simulink model "FUZZY_deg_neurospora_model_leloup"  (R2015a)
settings: Solver=ode4  StartTime=0.0  StopTime=72  FixedStep=0.01  RelTol=1e-3
values from neighbouring files (symbols this model uses):
  daynight_on = 0    [ALL_neurospora_init.m]    (also in ALL_neurospora_sim_run.m; FUZZY_deg_neurospora_init.m; FUZZY_deg_neurospora_sim_run.m; FUZZY_tsc_neurospora_init.m)
  k_1 = 0.5    [ALL_neurospora_init.m]    (also in FUZZY_deg_neurospora_init.m; FUZZY_tsc_neurospora_init.m; FUZZY_tsc_tsl_neurospora_init.m; FUZZY_tsl_neurospora_init.m)
  k_2 = 0.6    [ALL_neurospora_init.m]    (also in FUZZY_deg_neurospora_init.m; FUZZY_tsc_neurospora_init.m; FUZZY_tsc_tsl_neurospora_init.m; FUZZY_tsl_neurospora_init.m)
  K_I = 1    [ALL_neurospora_init.m]    (also in FUZZY_deg_neurospora_init.m; FUZZY_tsc_neurospora_init.m; FUZZY_tsc_tsl_neurospora_init.m; FUZZY_tsl_neurospora_init.m)
  k_s = 0.5    [ALL_neurospora_init.m]    (also in FUZZY_deg_neurospora_init.m; FUZZY_tsc_neurospora_init.m; FUZZY_tsc_tsl_neurospora_init.m; FUZZY_tsl_neurospora_init.m)
  n = 4    [ALL_neurospora_init.m]    (also in FUZZY_deg_neurospora_init.m; FUZZY_tsc_neurospora_init.m; FUZZY_tsc_tsl_neurospora_init.m; FUZZY_tsl_neurospora_init.m)
libraries: fuzblock x2
settings Model: Creator=jureb  LastModifiedBy=jureb

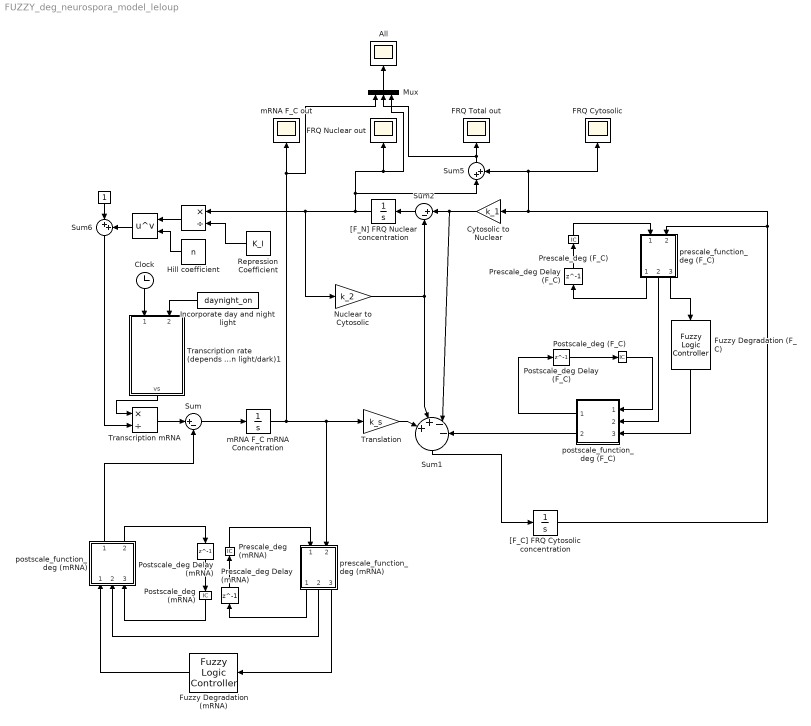
== system FUZZY_deg_neurospora_model_leloup ==
  " " : Math  Operator=pow  SaturateOnIntegerOverflow=on
  " " : Product  Inputs=*/
  "          " : Constant
  All : Scope
      settings: TimeRange=71.999776  YMin=0  YMax=9  SaveName=All
  Clock : Clock
  Cytosolic to Nuclear : Gain  Gain=k_1
  FRQ Cytosolic : Scope
      settings: TimeRange=71.999776  YMin=0.5  YMax=10  SaveName=F_C2
  FRQ Nuclear out : Scope
      settings: TimeRange=71.999776  YMin=0  YMax=4.5  SaveName=F_N
  FRQ Total out : Scope
      settings: TimeRange=71.999776  YMin=0.5  YMax=10  SaveName=F_FL_deg
  Fuzzy Degradation (F_C) : fuzblock/Fuzzy Logic  Controller  fis=deg
  Fuzzy Degradation (mRNA) : fuzblock/Fuzzy Logic  Controller  fis=deg
  Hill coefficient : Constant  Value=n
  Incorporate day and night light : Constant  Value=daynight_on
  Mux : Mux  Inputs=3
  Nuclear to Cytosolic : Gain  Gain=k_2
  Postscale_deg (F_C) : InitialCondition  Value=2
  Postscale_deg (mRNA) : InitialCondition  Value=0.5
  Postscale_deg Delay (F_C) : Delay  DelayLength=1  InitialCondition=1
  Postscale_deg Delay (mRNA) : Delay  DelayLength=1  InitialCondition=1
  Prescale_deg (F_C) : InitialCondition  Value=4
  Prescale_deg (mRNA) : InitialCondition  Value=4
  Prescale_deg Delay (F_C) : Delay  DelayLength=1  InitialCondition=1  UseCircularBuffer=on
  Prescale_deg Delay (mRNA) : Delay  DelayLength=1  InitialCondition=1  UseCircularBuffer=on
  Repression Coefficient : Constant  Value=K_I
  Sum : Sum  Inputs=|+-
  Sum1 : Sum  Inputs=|+|+|-|-
  Sum2 : Sum  Inputs=|+-
  Sum5 : Sum  Inputs=|++
  Sum6 : Sum  Inputs=|++
  Transcription mRNA : Product  Inputs=*/
  Transcription rate (depends on light/dark)1 : MATLAB Function  TreatAsAtomicUnit=on
  Translation : Gain  Gain=k_s
  "[F_C] FRQ Cytosolic concentration " : Integrator  InitialCondition=1
  "[F_N] FRQ Nuclear concentration" : Integrator  InitialCondition=1
  mRNA F_C mRNA Concentration : Integrator  InitialCondition=1  LowerSaturationLimit=0
  mRNA F_C out : Scope
      settings: TimeRange=71.999776  YMin=0  YMax=6  SaveName=mRNA
  postscale_function_deg (F_C) : MATLAB Function  TreatAsAtomicUnit=on
  postscale_function_deg (mRNA) : MATLAB Function  TreatAsAtomicUnit=on
  prescale_function_deg (F_C) : MATLAB Function  TreatAsAtomicUnit=on
  prescale_function_deg (mRNA) : MATLAB Function  TreatAsAtomicUnit=on
  wires:
  Sum6/1 -> Transcription mRNA/2
  "          "/1 -> Sum6/1
  Transcription mRNA/1 -> Sum/1
  " "/1 -> Sum6/2
  Hill coefficient/1 -> " "/2
  Sum/1 -> mRNA F_C mRNA Concentration/1
  " "/1 -> " "/1
  "[F_N] FRQ Nuclear concentration"/1 -> " "/1, Nuclear to Cytosolic/1, Mux/3, FRQ Nuclear out/1, Sum5/1
  Repression Coefficient/1 -> " "/2
  Sum1/1 -> "[F_C] FRQ Cytosolic concentration "/1
  Cytosolic to Nuclear/1 -> Sum1/3, Sum2/1
  Sum2/1 -> "[F_N] FRQ Nuclear concentration"/1
  Nuclear to Cytosolic/1 -> Sum1/2, Sum2/2
  Translation/1 -> Sum1/1
  Mux/1 -> All/1
  Clock/1 -> Transcription rate (depends on light/dark)1/1(sim_time)
  Transcription rate (depends on light/dark)1/1(vs) -> Transcription mRNA/1
  Incorporate day and night light/1 -> Transcription rate (depends on light/dark)1/2(daynight_on)
  Sum5/1 -> Mux/2, FRQ Total out/1
  Postscale_deg (mRNA)/1 -> postscale_function_deg (mRNA)/3(postscale_in)
  postscale_function_deg (mRNA)/2(postscale_out) -> Postscale_deg Delay (mRNA)/1
  Postscale_deg Delay (mRNA)/1 -> Postscale_deg (mRNA)/1
  Fuzzy Degradation (mRNA)/1 -> postscale_function_deg (mRNA)/1(output)
  prescale_function_deg (mRNA)/1(prescale_out) -> Prescale_deg Delay (mRNA)/1
  Prescale_deg (mRNA)/1 -> prescale_function_deg (mRNA)/1(prescale_in)
  Prescale_deg Delay (mRNA)/1 -> Prescale_deg (mRNA)/1
  prescale_function_deg (mRNA)/3(input_prescaled) -> Fuzzy Degradation (mRNA)/1
  prescale_function_deg (mRNA)/2(prescale_changed) -> postscale_function_deg (mRNA)/2(prescale_changed)
  mRNA F_C mRNA Concentration/1 -> Mux/1, mRNA F_C out/1, Translation/1, prescale_function_deg (mRNA)/2(input)
  postscale_function_deg (mRNA)/1(output_postscaled) -> Sum/2
  "[F_C] FRQ Cytosolic concentration "/1 -> prescale_function_deg (F_C)/2(input), Sum5/2, FRQ Cytosolic/1, Cytosolic to Nuclear/1
  Postscale_deg (F_C)/1 -> postscale_function_deg (F_C)/1(postscale_in)
  postscale_function_deg (F_C)/1(postscale_out) -> Postscale_deg Delay (F_C)/1
  Postscale_deg Delay (F_C)/1 -> Postscale_deg (F_C)/1
  Fuzzy Degradation (F_C)/1 -> postscale_function_deg (F_C)/3(output)
  postscale_function_deg (F_C)/2(output_postscaled) -> Sum1/4
  prescale_function_deg (F_C)/1(prescale_out) -> Prescale_deg Delay (F_C)/1
  Prescale_deg (F_C)/1 -> prescale_function_deg (F_C)/1(prescale_in)
  Prescale_deg Delay (F_C)/1 -> Prescale_deg (F_C)/1
  prescale_function_deg (F_C)/3(input_prescaled) -> Fuzzy Degradation (F_C)/1
  prescale_function_deg (F_C)/2(prescale_changed) -> postscale_function_deg (F_C)/2(prescale_changed)

== matlab function FUZZY_deg_neurospora_model_leloup/Transcription rate (depends on light//dark)1 ==
  data: sim_time input; vs output; daynight_on input
function vs = day_night(sim_time,daynight_on)

vs_day = 2;
vs_night = 1.6;

if daynight_on == 1
    if ((sim_time > 0 && sim_time < 12) || (sim_time > 24 && sim_time < 36) || (sim_time > 48 && sim_time < 60)) % DAY
        vs = vs_day;
    else % NIGHT
        vs = vs_night;
    end
else % NO DIFFERENTIATION BETWEEN NIGHT AND DAY
    vs = vs_night;
end

== matlab function FUZZY_deg_neurospora_model_leloup/postscale_function_deg (mRNA) ==
  data: output input; prescale_changed input; output_postscaled output; postscale_in input; postscale_out output
function [output_postscaled, postscale_out] = postscale(output,prescale_changed, postscale_in)

postscale_out = postscale_in;
multiplier = 1.01;

if (prescale_changed == 1)
    postscale_out = postscale_out*multiplier;
end

output_postscaled = output*postscale_out;

== matlab function FUZZY_deg_neurospora_model_leloup/postscale_function_deg (F_C) ==
  data: postscale_in input; prescale_changed input; postscale_out output; output input; output_postscaled output
function [postscale_out, output_postscaled] = postscale(postscale_in,prescale_changed, output)

postscale_out = postscale_in;
multiplier = 1.01;

if (prescale_changed == 1)
    postscale_out = postscale_out*multiplier;
end

output_postscaled = output*postscale_out;

== matlab function FUZZY_deg_neurospora_model_leloup/prescale_function_deg (mRNA) ==
  data: prescale_in input; prescale_out output; prescale_changed output; input input; input_prescaled output
function [prescale_out, prescale_changed, input_prescaled] = prescale(prescale_in, input)

prescale_out = prescale_in;
multiplier = 1.01;
prescale_changed = 0;

if (input >= 0.9*prescale_in)
    prescale_out = prescale_in*multiplier;
    prescale_changed = 1;
end

input_prescaled = input/prescale_out;

== matlab function FUZZY_deg_neurospora_model_leloup/prescale_function_deg (F_C) ==
  data: prescale_in input; prescale_out output; prescale_changed output; input input; input_prescaled output
function [prescale_out, prescale_changed, input_prescaled] = prescale(prescale_in, input)

prescale_out = prescale_in;
multiplier = 1.01;
prescale_changed = 0;

if (input >= 0.9*prescale_in)
    prescale_out = prescale_in*multiplier;
    prescale_changed = 1;
end

input_prescaled = input/prescale_out;
